simulink model "base_model_lqeH"  (R2020b)
settings: Solver=ode1  StartTime=0  StopTime=1150  FixedStep=0.1  RelTol=1e-3
libraries: simulink_extras x33
(part 2 of 3)

== matlab function base_model_lqeH/FormZ ==
  data: satInfo output size=[4,8]; satVisible input uint8 size=1; satCount input size=1; satCountPreset input; satVisibleFlag_GNSS input size=32; psdRange_sat input size=32; psdRange_INS input size=32; psdVel_INS input size=32; psdVel_sat input size=32; satNum output size=1; psdRange_INS_short output size=8; psdRange_GNSS_short output size=[8,1]; satVisibleFlag_INS input; satPosVel input; satPosVel_short output; dPsdRange input; sigmPsdRange output; satIDvis output uint8; satAzimutVis output; satEleavtionVis output; satAzimut input; satElevation input
function [satInfo, satNum, psdRange_INS_short, psdRange_GNSS_short, satPosVel_short, sigmPsdRange, satIDvis, satAzimutVis, satEleavtionVis] = ...
    getDGSK(satVisible, satCount, satCountPreset, satVisibleFlag_GNSS, psdRange_sat, ... 
    psdRange_INS,psdVel_INS, psdVel_sat, satVisibleFlag_INS, satPosVel, dPsdRange, satAzimut, satElevation)

    satCountPreset_fix = 20;
    
    satInfo             = zeros(4,8);
    psdRange_INS_short  = zeros(8,1);
    psdRange_GNSS_short = zeros(8,1);
    satPosVel_short     = zeros(6,8);
    sigmPsdRange        = zeros(8,1);
    
    satIDvis            = uint8(zeros(8,1));
    satAzimutVis        = zeros(8,1);
    satEleavtionVis     = zeros(8,1);
    
    satNum  = uint8(0);
    d_psdRange = 0;
    d_psdVel   = 0;
    for satID = 1:satCount
        
        if satVisibleFlag_GNSS(satID) == 1 && satVisibleFlag_INS(satID) == 1
            if satNum < satCountPreset
                satNum = satNum + 1;
            end
            d_psdRange = psdRange_INS(satID) - psdRange_sat(satID);
            d_psdVel   = psdVel_INS(satID)   - psdVel_sat(satID);
            
            satInfo(4,satNum) = psdRange_INS(satID);
            satIDvis(satNum)  = uint8(satID);
            
            
            satInfo(1,satNum) = satID;
            satInfo(2,satNum) = d_psdRange;
            satInfo(3,satNum) = d_psdVel;
            
            satAzimutVis(satNum)    = satAzimut(satID);
            satEleavtionVis(satNum) = satElevation(satID);
            
            satPosVel_short(:,satNum) = satPosVel(:,satID);
            
            sigmPsdRange(satNum) = dPsdRange(satID);
           
            
            psdRange_INS_short(satNum)  = psdRange_INS(satID);
            psdRange_GNSS_short(satNum) = psdRange_sat(satID);
        end      
    end
end

== matlab function base_model_lqeH/GNNS_freq_imitetor ==
  data: satNum_AV input size=1; satInfo output size=[4,8]; satInfo_AV input size=[4,8]; time_shift input size=1; satNum output uint8 size=1; timeDelay output size=1; frameAvalible_GNSS output uint8 size=1; satPosVel_AV input; satPosVel output; tStart input; tEnd input
function [satInfo, satNum, timeDelay, frameAvalible_GNSS,satPosVel]= getDGSK(satNum_AV, satInfo_AV, time_shift, satPosVel_AV, tStart, tEnd)

    satInfo   = zeros(4,8);
    satNum    = uint8(0);
    timeDelay = 0;
    satPosVel = zeros(6,8);

    GNSS_delay = 1;
    frameAvalible_GNSS = uint8(0);

    persistent time satInfo_mem satNum_mem satPosVel_mem timeInit

    if isempty(time)
        time = 0;
        timeInit = 0;
        
        satInfo_mem   = zeros(4,8);
        satNum_mem    = uint8(0);
        satPosVel_mem = zeros(6,8);
        
    end
    
    if timeInit > tStart
    
        if time > GNSS_delay
            satInfo_mem   = satInfo_AV  ; 
            satNum_mem    = satNum_AV   ;
            satPosVel_mem = satPosVel_AV;
            timeDelay     = time        ;
            time = 0;
            frameAvalible_GNSS = uint8(1);
        end

        timeDelay = GNSS_delay  ;
        satInfo   = satInfo_mem  ; 
        satNum    = satNum_mem   ;
        satPosVel = satPosVel_mem;

    %     satInfo(satErrNum) = satInfo(satErrNum) + psdErr;
    %     satInfo(1:3) = satInfo(1:3) + psdErr;

        time = time + time_shift;
    end
    timeInit = timeInit + time_shift;
end

== matlab function base_model_lqeH/GNSS_receiver_imitator6 ==
  data: alpha input; dyaw output; beta input; gamma input; heading input; pitch input; roll input; dpitch output; droll output; matr_CORR output
function [dyaw, dpitch,droll, matr_CORR] = GNSS_receiver_imitator (alpha, beta, gamma, heading, pitch, roll)

yaw = heading;
matr_CORR = zeros(3,3);
matrix = [sin(yaw)*tan(pitch), cos(yaw)*tan(pitch), -1;
          cos(yaw),           -sin(yaw),             0;
          sin(yaw)/cos(pitch), cos(yaw)/cos(pitch),  0];

dangles = [0;0;0];       

dangles = matrix*[alpha;beta;gamma];

dyaw   =  dangles(1);
dpitch =  dangles(2);
droll  =  dangles(3);
% 
% 
fix_heading = heading - dyaw;          
fix_pitch   = pitch   - dpitch;          
fix_roll    = roll    - droll;
% 
% matr_CORR = [ fix_heading,0,0;...
%              fix_pitch,0,0;...
%              fix_roll,0,0];
      
% matr_CORR =  [0 ,  gamma,-beta;...
%              -gamma, 0,  alpha;...
%               beta, -alpha, 0]; 

matr_CORR =  [ 0,       dyaw, -droll; ...
              -dyaw,    0,     dpitch;...
               droll, -dpitch, 0];

% matr_CORR =  [ dyaw, 0,      0; ...
%                0,    dpitch, 0;...
%                0,    0,      droll];







% if lqe_ctrl(1) == 1
%     mean_heading = circshift(mean_heading,-1);
%     mean_pitch   = circshift(mean_pitch,-1);
%     mean_roll    = circshift(mean_roll,-1);
% 
%     mean_heading(1) = dyaw;
%     mean_pitch(1)   = dpitch;
%     mean_roll(1)    = droll;
% 
% 
% end
% 
%     dyaw   = mean(mean_heading);
%     dpitch = mean(mean_pitch);
%     droll  = mean(mean_roll);


end

== matlab function base_model_lqeH/seter1 ==
  data: signal output size=1; time_shift input
function signal  = slowData(time_shift)
  
    persistent time_mem

    if isempty(time_mem)
        time_mem = 0;
    end
    
    signal = 0;
    time_mem = time_mem + time_shift;
    
    if time_mem >= 1
        signal = 1;
        time_mem = 0;
    end
    
end

== matlab function base_model_lqeH/DOPS ==
  data: PDOP output size=1; satPosVel input; HDOP output size=1; VDOP output size=1; TDOP output; satInfo input; psdRange_GNSS_short input size=[8,1]; satCountPreset input; posObj input; DOP output
function [PDOP, HDOP, VDOP,TDOP,DOP] = ...
    DOPS(satPosVel, satInfo, psdRange_GNSS_short, satCountPreset, posObj)

    PDOP = 0;
    HDOP = 0;
    VDOP = 0;
    TDOP = 0;
    DOP  = 0;
    matrixH = zeros(satCountPreset, 4);
    
%     satNum = 0;
    
    for ii = 1:satCountPreset
        if ii < length(satInfo(1,:))
            matrixH(ii, 1) = (satPosVel(1,ii) - posObj(1)) / psdRange_GNSS_short(ii);
            matrixH(ii, 2) = (satPosVel(2,ii) - posObj(2)) / psdRange_GNSS_short(ii);
            matrixH(ii, 3) = (satPosVel(3,ii) - posObj(3)) / psdRange_GNSS_short(ii);
            matrixH(ii, 4) = 1;
        end
    end
    
    Krt_2 = trace(inv(matrixH' * matrixH));
    
    
    Kr_2 = Krt_2 * 4/5;
    Kh_2 = Kr_2 * (1/((1/1.5 + 1)^2));
    
    DOP  = sqrt(Krt_2) ;
    PDOP = sqrt(Kr_2)  ; 
    TDOP = sqrt(Kr_2)/2;
    
    HDOP = sqrt(Kh_2)  ;
    VDOP = sqrt(Kh_2)*1.5;
    
    
    if  isnan(DOP)
        zz = 1;
    end
    
    
    
end

== matlab function base_model_lqeH/seter2 ==
  data: signal output size=1; time_shift input
function signal  = slowData(time_shift)
  
    persistent time_mem

    if isempty(time_mem)
        time_mem = 0;
    end
    
    signal = 0;
    time_mem = time_mem + time_shift;
    
    if time_mem >= 1
        signal = 1;
        time_mem = 0;
    end
    
end

== matlab function base_model_lqeH/Ve_err 1 ==
  data: data_out output size=1; data_in input; ctrl input
function data_out  = slowData(data_in, ctrl)
  
    persistent data_mem

    if isempty(data_mem)
        data_mem = data_in;
    end
    
    if ctrl == 1
        data_mem = data_in;
    end
    
    data_out = data_mem;
    
    
end

== matlab function base_model_lqeH/Fuck matlab5 ==
  data: satNum output; satVisible input; satIDs_fix output; psdRange_INSvis_fix output; psdRange_GNSSvis_fix output; satIDs input; baseSatID output; psdRange_INSvis input; psdRange_GNSSvis input; satCountPreset input
function [satNum, satIDs_fix,psdRange_INSvis_fix, psdRange_GNSSvis_fix, baseSatID]=  integrity_control(satVisible, satIDs, psdRange_INSvis, psdRange_GNSSvis, satCountPreset)
    
    %ограничивание числа спутников до satCountPreset = 8
    
    satIDs_fix           = zeros(8,1);
    psdRange_INSvis_fix  = zeros(8,1);
    psdRange_GNSSvis_fix = zeros(8,1);
    
    satNum = min([satVisible, satCountPreset]);
    
    for ii = 1:satVisible
        if ii <= satCountPreset
            satIDs_fix(ii) = satIDs(ii);
            psdRange_INSvis_fix (ii) = psdRange_INSvis(ii);
            psdRange_GNSSvis_fix(ii) = psdRange_GNSSvis(ii);
        end
    end

    baseSatID = satIDs(1);


end

== matlab function base_model_lqeH/Fuck matlab6 ==
  data: satAv output; satVisible input; satID_shrt input; satID_IC input
function satAv =  integrity_control(satVisible, satID_shrt, satID_IC)
    
    satAv = ones(8,1);
    persistent aa 
    if isempty(aa)
        aa = 0;
    end
        
    for ii = 1:8
        jj = find(satID_IC(ii) == satID_shrt);
        if ~isempty(jj)
            satAv(jj) = 0;
        end
    end


end

== matlab function base_model_lqeH/Fuck matlab7 ==
  data: psdRMiss output; size input
function psdRMiss =  integrity_control(size)
    
    psdRMiss = ones(8,1) .* size;

    
end

== matlab function base_model_lqeH/GNSS_integrity_control1 ==
  data: satNum input uint8 size=1; satID_in input; satAzimut_in input; satElevation_in input; psdRangeINS_in input; psdRangeGNSS_in input; baseSatID input uint8 size=1; satID_IC output uint8; intCtrl_status output uint8 size=1; lqe_F input; lqe_P input; lqe_L input; lqe_Q input; posObjINS input size=3; satPosVel input; lat input; lon input; alt input; disp_SatPos input; frameAvalible input; fastCritLevel output; fastLevel output; slowCritLevel output; satStartTime input; time_shift input; sensitivity input size=[4,1]; z_level output; z_crout output

function [satID_IC, intCtrl_status, fastCritLevel, fastLevel, slowCritLevel,...
          z_level, z_crout]=  integrity_control(satNum, satID_in, satAzimut_in, satElevation_in, ...
                                                         psdRangeINS_in, psdRangeGNSS_in, baseSatID,...                                                     
                                                         lqe_F, lqe_P, lqe_L, lqe_Q, posObjINS, satPosVel, lat, lon, alt, disp_SatPos, frameAvalible, satStartTime, time_shift, sensitivity)

    persistent intCtrl qq time
%--------------------------------------------------------------------------
%Константы
    disp_SatVel = 0.03;
    
    
    
    if isempty(intCtrl)
               
        qq = 0;
        time = 0;
        slowWindow = 600;% set max for code generation
        satLimit   = 8;
        
%         intCtrl.sensitivity = zeros(3,1);
        intCtrl.slowSensitivity = sensitivity(3);
        
        intCtrl.fastInit = uint8(0);
        intCtrl.psdRangeFast = zeros(satLimit,3);
        intCtrl.fastSatList = zeros(satLimit,1);
        
        
        intCtrl.slowInit = uint8(0);
        intCtrl.psdRangeSlow = ones(slowWindow,satLimit);
        intCtrl.slowSatList  = zeros(satLimit,1);
        
        intCtrl.probSatID = uint8(zeros(satLimit,1));
        intCtrl.moniSatID = uint8(zeros(satLimit,1));
        
        intCtrl.probSatNum = uint8(0);
        intCtrl.moniSatNum = uint8(0);
        
        intCtrl.baseSatID = uint8(0);
        
        intCtrl.satLossFrame     = zeros(satLimit,2); %Строка 1 не задейстоввана?
        intCtrl.satLossFrameAlow = uint8(10);
        
        intCtrl.slowMean = zeros(satLimit,2);
        intCtrl.slowDisp = zeros(satLimit,1);
        
        intCtrl.fastExpt = zeros(satLimit,1);%Не задействовано
        
        intCtrl.fastExptCriteria = zeros(satLimit,2);
        
        intCtrl.criteriaScale = ones(2,1) .* [sensitivity(1); sensitivity(2)]; 
        
        intCtrl.slowWindow      = slowWindow;
        intCtrl.slowWindow_size = sensitivity(4);
        intCtrl.satLimit        = satLimit;
    end
%--------------------------------------------------------------------------
%Объявление выходых параметров 
    satID_IC       = uint8(zeros(8 ,1));%uint8(zeros(intCtrl.satLimit ,1));
    fastCritLevel  =       zeros(8,1);%zeros(intCtrl.satLimit ,1);
    fastLevel      =       zeros(8,1);%zeros(intCtrl.satLimit ,1);
    slowCritLevel  =       zeros(8,1);%zeros(intCtrl.satLimit ,1);
    intCtrl_status =       uint8(1); %%uint8(1); %
    z_crout        =       zeros(1,1);%zeros(1,1);
    z_level        =       zeros(8,1);%zeros(intCtrl.satLimit ,1);
    
%--------------------------------------------------------------------------
%Костыль для подержания много спутников (Если всегда +- 8 но подскакивает до 12)

    satID        = uint8(zeros(intCtrl.satLimit,1));
    satAzimut    =       zeros(intCtrl.satLimit,1);
    satElevation =       zeros(intCtrl.satLimit,1);
    psdRangeINS  =       zeros(intCtrl.satLimit,1);
    psdRangeGNSS =       zeros(intCtrl.satLimit,1);
    
    for ii = 1:satNum
        satID(ii)        = satID_in(ii);
        satAzimut(ii)    = satAzimut_in(ii);
        satElevation(ii) = satElevation_in(ii);
        psdRangeINS(ii)  = psdRangeINS_in(ii);
        psdRangeGNSS(ii) = psdRangeGNSS_in(ii);
    end

%--------------------------------------------------------------------------  
%Обновление ID базового спутника
    intCtrl.baseSatID = baseSatID;
%--------------------------------------------------------------------------
%Счетчик пропущенных измерений НКА. Для "рабочих" НКА, счетчик обнуляется 
    intCtrl.satLossFrame(:,2) = intCtrl.satLossFrame(:,2) + 1;
    for ii = 1:satNum
        if find(satID(ii) == intCtrl.satLossFrame(:,1))
            intCtrl.satLossFrame(ii,2) = 0;
        end
    end
%--------------------------------------------------------------------------
    if frameAvalible == 1                                                  %Ждать поступления измерения псевдодальности
                                                                           %Быстрый цикл  
%                                                                          Набор информации (первых и вторых разностей)
        intCtrl = fastCircle (intCtrl, satNum, satID, psdRangeGNSS, psdRangeINS, disp_SatPos,...
                              lqe_F, lqe_P, lqe_L, lqe_Q, lat, lon, alt, posObjINS, satPosVel, disp_SatVel);
                                                                            %Набор информации (первых разностей)
                                                                           %Проверка по критерию
        probSatCount = 0;
        %intCtrl.probSatID = uint8(zeros(intCtrl.satLimit,1));%
        intCtrl.probSatID = uint8(zeros(8,1));
        for ii = 1:satNum
            if abs(intCtrl.psdRangeFast(ii,3)) >= (intCtrl.fastExptCriteria(ii))
                probSatCount = probSatCount + 1;
                intCtrl.probSatID(probSatCount) = satID(ii);
            end
        end
                                                                            %Медленный цикл  
                                                                            %Набор информации (вторых разностей и среднего)
    intCtrl = slowCircleLogic(intCtrl, satNum, satID, psdRangeGNSS, psdRangeINS);
%     
    
    for ii = 1:satNum
        baseMean = 0;
        baseDisp = intCtrl.slowDisp(ii);
%         alpha = intCtrl.slowSensitivity;
%         Z = (intCtrl.slowMean(ii) -  baseMean) ./ sqrt(intCtrl.slowDisp(ii) * 2/intCtrl.slowWindow(1:intCtrl.slowWindow_size));
%may be ERROR        
        Z = (intCtrl.slowMean(ii) -  baseMean) ./ sqrt(intCtrl.slowDisp(ii) * 2/intCtrl.slowWindow_size);
%         Z_criteria = tinv(1 - intCtrl.slowSensitivity, intCtrl.slowWindow(1:intCtrl.slowWindow_size) - 2 - 1);
        Z_criteria = tinv(intCtrl.slowSensitivity, intCtrl.slowWindow_size - 2 - 1);%(1:intCtrl.slowWindow_size)
        z_level(ii) = abs(Z);
        z_crout = Z_criteria;
   %Slow circle decision-making segment
        if abs(Z) >= Z_criteria
            jj = find(satID(ii) == intCtrl.probSatID);
            if length(jj) == 0
                probSatCount = probSatCount + 1;        
                intCtrl.probSatID(probSatCount) = satID(ii);  
                qq = qq + 1;
                if qq == 900
                    tt = 1;
                end
            end
        end
    end
    
    end
    
fastLevel     = abs(intCtrl.psdRangeFast(:,3));    
fastCritLevel = intCtrl.fastExptCriteria(:,1);
slowCritLevel = abs(intCtrl.slowMean(:,1));
% z_level = abs(Z);
% z_crout = Z_criteria;

%--------------------------------------------------------------------------
    
%--------------------------------------------------------------------------
                                                                            %Отбор спутников и формирование выходной информации
                                                                     
    id = 0;
    intCtrl_status = uint8(1);% 1 - IC pass; 0 - IC fault
    time = time + time_shift;
%     if time > (satStartTime + intCtrl.slowWindow(1:intCtrl.slowWindow_size) * 4) 
    if time > (satStartTime + intCtrl.slowWindow_size * 4)%(1:intCtrl.slowWindow_size)
        for ii = 1:satNum
            if find(satID(ii) == intCtrl.probSatID)
                id = id + 1;
                satID_IC(id) = satID(ii);
            end
        end
        if satNum - id <= 4  
            intCtrl_status = uint8(0);
        end
    end
    
end


%==========================================================================
function [D_rho, D_rho_dot] = fastCriteriaMath( a,e2,C,Ro_mark,R_tp,disp_SatPos_mem, ...
                                    ii,lat,lon,alt, psdRange,posObj, satPosVel,...
                                    disp_SatPos, disp_SatVel)
        
        
        dPsdRange_dLambda =  (1/psdRange(ii)) * (Ro_mark + alt)*cos(lat)*...
                                                (sin(lon)*(satPosVel(1,ii) - posObj(1)) - ...
                                                 cos(lon)*(satPosVel(2,ii) - posObj(2)));

        dPsdRange_dphi    =  (1/psdRange(ii))   * ...
                              ((satPosVel(1,ii) - posObj(1)) * (- cos(lon) * cos(lat) * R_tp + (Ro_mark + alt) * cos(lon) * sin(lat)) + ...%dRz_dLat
                               (satPosVel(2,ii) - posObj(2)) * (- sin(lon) * cos(lat) * R_tp + (Ro_mark + alt) * sin(lon) * sin(lat)) + ...%dRz_dLat
                               (satPosVel(3,ii) - posObj(3)) * (- (1 - e2) * sin(lat) * R_tp - ((1 - e2) * Ro_mark + alt) * cos(lat)));    %dRz_dLat

        dPsdVel_dot_dVe   =  (1/psdRange(ii)) * (...
                                sin(lon) * (satPosVel(1,ii) - posObj(1)) - ...
                                cos(lon) * (satPosVel(2,ii) - posObj(2)));

        dPsdVel_dot_dVn   =  (1/psdRange(ii)) * (...
                                cos(lon)*sin(lat)*(satPosVel(1,ii) - posObj(1)) + ...
                                sin(lon)*sin(lat)*(satPosVel(2,ii) - posObj(2)) - ...
                                cos(lat)*         (satPosVel(3,ii) - posObj(3)));

        dPsdRange_dAlt    = (-1/psdRange(ii))* (...
                                cos(lat)*cos(lon)*(satPosVel(1,ii) - posObj(1)) + ...
                                cos(lat)*sin(lon)*(satPosVel(2,ii) - posObj(2)) + ...
                                sin(lat)*         (satPosVel(3,ii) - posObj(3)));
%--------------------------------------------------------------------------
%Формирование дисперсий
        dPsdVel_dot_dVh   = (-1/psdRange(ii))* (...
                                cos(lon)*cos(lat)*(satPosVel(1,ii) - posObj(1)) + ...
                                sin(lon)*cos(lat)*(satPosVel(2,ii) - posObj(2)) + ...
                                sin(lat)*         (satPosVel(3,ii) - posObj(3)));
%--------------------------------------------------------------------------
%Пересчет из радиан в метры
                            
        ro_1 = a*(1-e2)/(1-e2*sin(lat)^2)^(3/2) + alt;
        ro_2 = a*(1-e2*sin(lat)^2)^(-1/2) + alt;                      
        dPsdRange_dLambda =  (1/(ro_2 * cos(lat))) * dPsdRange_dLambda;
        dPsdRange_dphi    =  (1/ro_1) * dPsdRange_dphi;                 
%--------------------------------------------------------------------------
        D_hor = sum(abs([dPsdRange_dLambda, dPsdRange_dphi ]) * [C(1,1), C(1,2) ;...
                                                            C(2,1), C(2,2)]);
        D_vel = sum(abs([dPsdVel_dot_dVe,   dPsdVel_dot_dVn]) * [C(3,3), C(3,4) ;...
                                                            C(4,3), C(4,4)]);    
                                                        
        D_alt  = abs(dPsdRange_dAlt)  * C(20,20);
        D_vAlt = abs(dPsdVel_dot_dVh) * C(21,21);


        D_rho     = D_hor + D_alt  + disp_SatPos + disp_SatPos_mem;
        D_rho_dot = D_vel + D_vAlt + 2*disp_SatVel;

end



function intCtrl = fastCircle(intCtrl, satNum, satID, psdRangeGNSS, psdRangeINS, disp_SatPos,...
                              lqe_F, lqe_P, lqe_L, lqe_Q, lat, lon, alt, posObjINS, satPosVel, disp_SatVel)
    
    persistent disp_SatPos_mem

    if isempty(disp_SatPos_mem)
        disp_SatPos_mem = zeros(size(disp_SatPos));
        disp_SatPos_mem = disp_SatPos;
    end

%--------------------------------------------------------------------------
%Константы    
    a = 6378136;
    e2 = 0.0066943662;
%--------------------------------------------------------------------------
%Матрица связи С (?)        
    C = lqe_F*lqe_P*lqe_F' + lqe_L*lqe_Q*lqe_L' + lqe_P + 2*lqe_F*lqe_P;
    Ro_mark = a / sqrt(1 - e2*(sin(lat))^2);
%--------------------------------------------------------------------------
%Коэффициенты (направляющие косинусы). Аналагично матрице связи Н (ЖСК)        
    
    dRz_dLat = a*e2*cos(lat)*sin(lat) / ((1 - e2*sin(lat)^2)^(3/2));
    R_tp     = sin(lat)*(a + alt) - cos(lat)*dRz_dLat;  

    if intCtrl.fastInit == 0
        for ii = 1:satNum
            intCtrl.psdRangeFast(ii, 1) = 1;%(psdRangeGNSS(ii) - psdRangeGNSS(intCtrl.baseSatID));
            intCtrl.psdRangeFast(ii, 2) = intCtrl.psdRangeFast(ii, 1);
            intCtrl.fastSatList(ii)     = satID(ii);
            intCtrl.fastInit            = uint8(1); 
        end
    end


    for ii = 1:satNum
        sID = find(satID(ii) == intCtrl.fastSatList);%Был ли этот спутник раньше
        if ~isempty(sID) %Если этот спутник уже есть и обрабатывается 
            
            thirdDifference_previous = intCtrl.psdRangeFast(sID, 1);
            intCtrl.psdRangeFast(sID, 1) = psdRangeGNSS(sID) - psdRangeINS(sID);
            intCtrl.psdRangeFast(sID, 3) = intCtrl.psdRangeFast(sID, 1) - thirdDifference_previous;                                               
%             
            [D_rho, D_rho_dot] = fastCriteriaMath( a,          e2,        C,  Ro_mark,      R_tp, disp_SatPos_mem(ii), ...
                                                  ii,      lat,      lon,       alt, psdRangeINS,   posObjINS, satPosVel, disp_SatPos(ii), disp_SatVel);
                                                  
            intCtrl.fastExptCriteria(sID,1) = intCtrl.criteriaScale(1) * sqrt(abs(D_rho)    );
            intCtrl.fastExptCriteria(sID,2) = intCtrl.criteriaScale(2) * sqrt(abs(D_rho_dot));
        
        else % Если появился спутник
            if ii <= intCtrl.satLimit % Если не превышен лимит н спутники
                if length(find(intCtrl.fastSatList == 0)) ~= 0% Если есть слоты для спутников
                    %------Инициализация
                    sID = find(intCtrl.fastSatList == 0, 1,'first');% Вязть первый пустой слот
                    intCtrl.fastSatList (sID)    = satID(ii);% Записать ID нового спутника
                    
                    %--------------------------------------
                    %Замена на 3 разности
                            thirdDifference_previous = intCtrl.psdRangeFast(sID, 1);
                            intCtrl.psdRangeFast(sID, 1) = psdRangeGNSS(sID) - psdRangeINS(sID);
                            intCtrl.psdRangeFast(sID, 3) = intCtrl.psdRangeFast(sID, 1) - thirdDifference_previous;  
                    
                  
                    [D_rho, D_rho_dot] = fastCriteriaMath(   a,          e2,        C, dRz_dLat,      R_tp, disp_SatPos_mem(ii), ...
                                                            ii,      lat,      lon,       alt, psdRangeINS,   posObjINS, satPosVel, disp_SatPos(ii), disp_SatVel);                           
                    intCtrl.fastExptCriteria(sID,1) = intCtrl.criteriaScale(1) * sqrt(abs(D_rho)    );
                    intCtrl.fastExptCriteria(sID,2) = intCtrl.criteriaScale(2) * sqrt(abs(D_rho_dot));
                    
                else % Если нет слотов
                    jj = find(intCtrl.satLossFrame(:,2) >= intCtrl.satLossFrameAlow, 1, 'first');%Найти просрочку
                    if ~isempty(jj)% Если есть просроченые спутники
                    %------Инициализация
                        intCtrl.fastSatList(jj)     = satID(ii);
                    %--------------------------------------
                    %Замена на 3 разности
                            thirdDifference_previous = intCtrl.psdRangeFast(sID, 1);
                            intCtrl.psdRangeFast(sID, 1) = psdRangeGNSS(sID) - psdRangeINS(sID);
                            intCtrl.psdRangeFast(sID, 3) = intCtrl.psdRangeFast(sID, 1) - thirdDifference_previous; 
                        
                                   
                        [D_rho, D_rho_dot] = fastCriteriaMath(	 a,          e2,        C, dRz_dLat,       R_tp, disp_SatPos_mem(ii), ...
                                                                ii,      lat,      lon,       alt, psdRangeINS,   posObjINS, satPosVel, disp_SatPos(ii), disp_SatVel);
                                                  
                        intCtrl.fastExptCriteria(sID,1) = intCtrl.criteriaScale(1) * sqrt(abs(D_rho)    );
                        intCtrl.fastExptCriteria(sID,2) = intCtrl.criteriaScale(2) * sqrt(abs(D_rho_dot));
                    end
                end
            end
        end
        
        
    end
    
end








function intCtrl = slowCircleLogic(intCtrl, satNum, satID, psdRangeGNSS, psdRangeINS)

%--------------------------------------------------------------------------
%Инициализация
    if intCtrl.slowInit == 0
        for ii = 1:satNum
            intCtrl.slowSatList(ii)    = satID(ii);
%             intCtrl.psdRangeSlow(:,ii) = intCtrl.psdRangeSlow(:,ii) .*...
%                 ((psdRangeGNSS(ii)                   - psdRangeINS(ii))     ...
%                - (psdRangeGNSS(intCtrl.baseSatID) - psdRangeINS(intCtrl.baseSatID)));
        end
        intCtrl.slowInit = uint8(1);
    end
%--------------------------------------------------------------------------
%Медленный цикл
    for ii = 1:satNum
%         if find(satID(ii) ~= intCtrl.probSatID)
        if find(satID(ii) == intCtrl.slowSatList) %Если спутник уже был
            intCtrl = slowCircleAction(intCtrl, ii, psdRangeGNSS(ii), psdRangeINS(ii)); %обработка
        else 
            if length(find(intCtrl.slowSatList == 0)) ~= 0% Если есть слоты для спутников
                %------Инициализация
                sID = find(intCtrl.slowSatList == 0, 1,'first');% Взять первый пустой слот
                intCtrl.slowSatList(sID) = satID(ii);
                %max set only here
                intCtrl.psdRangeSlow((1:intCtrl.slowWindow_size),sID) = ones(uint16(intCtrl.slowWindow_size),1).*...
                                                 (psdRangeGNSS(ii)                - psdRangeINS(ii));% - ...
                                                  %(psdRangeGNSS(intCtrl.baseSatID) - psdRangeINS(intCtrl.baseSatID)));
                intCtrl = slowCircleAction(intCtrl, sID, psdRangeGNSS(ii), psdRangeINS(ii));
                fkngtest = 1;
            else % Если нет слотов
                jj = find(intCtrl.satLossFrame(:,2) >= intCtrl.satLossFrameAlow, 1, 'first');%Найти просрочку
                if ~isempty(jj)% Если есть просроченые спутники
                %------Инициализация
                    intCtrl.slowSatList(jj) = satID(ii);
                    intCtrl.psdRangeSlow((1:intCtrl.slowWindow_size),jj) = ones(uint16(intCtrl.slowWindow_size),1).*...
                                                    (psdRangeGNSS(ii)                - psdRangeINS(ii));
                    intCtrl = slowCircleAction(intCtrl, jj, psdRangeGNSS(ii), psdRangeINS(ii));
                end
            end
        end
            
            
            
            
            
%             if ii <= intCtrl.satLimit %Если не превышено количество спутников
%                 jj = find(intCtrl.satLossFrame(:,2) >= intCtrl.satLossFrameAlow, 1, 'first');% 
%                 intCtrl.slowSatList(jj) = satID(ii);
% 
%                 intCtrl.psdRangeSlow(:,jj) = ones(intCtrl.slowWindow(1:slowWindow_size),1).*...
%                                                 ((psdRangeGNSS(ii)                - psdRangeINS(ii))...
%                                                - (psdRangeGNSS(intCtrl.baseSatID) - psdRangeINS(intCtrl.baseSatID)));
% 
%                 intCtrl = slowCircleAction(intCtrl, jj, psdRangeGNSS, psdRangeINS);
%             end
%         end
%         end
    end
end

function intCtrl = slowCircleAction(intCtrl, id, psdRangeGNSS, psdRangeINS)

    intCtrl.psdRangeSlow(1:intCtrl.slowWindow_size,id) = circshift(intCtrl.psdRangeSlow(1:intCtrl.slowWindow_size,id),1);
    intCtrl.psdRangeSlow(1,id) = (psdRangeGNSS - psdRangeINS);
   %intCtrl.psdRangeSlow(1,id) = (psdRangeGNSS(id) - psdRangeINS(id)) - (psdRangeGNSS(intCtrl.baseSatID) - psdRangeINS(intCtrl.baseSatID));  
    intCtrl.psdRangeSlow(1,id) = intCtrl.psdRangeSlow(1,id) - intCtrl.slowMean(id,2);
    intCtrl.slowMean(id,2)     = (psdRangeGNSS - psdRangeINS);
    
    
    intCtrl.slowMean(id,1)= mean(intCtrl.psdRangeSlow(1:intCtrl.slowWindow_size,id));
    intCtrl.slowDisp(id)  =  std(intCtrl.psdRangeSlow(1:intCtrl.slowWindow_size,id));
end

== matlab function base_model_lqeH/Fuck matlab8 ==
  data: corruptValue output; tStart input; tp input; tEnd input; errSize input; corruptTimeStart input; corruptPSDError input; corruptErrorType input; dt input
function corruptValue = integrity_control(tStart, tp, tEnd, errSize,...
                    corruptTimeStart, corruptPSDError, corruptErrorType, dt)
%chouse psd error type
    persistent time
    if isempty(time)  
        time = 0;
    end
    corruptValue = 0;
    if time >= corruptTimeStart
        
        if corruptErrorType == 1
            corruptValue = corruptPSDError;
        elseif corruptErrorType == 2
            corruptValue = corruptPSDError * (time - corruptTimeStart);
        else
            corruptValue = 0;
        end
    end

    time = time + dt;


    % %--------------------------------------------------------------------------
    % if time > tStart && time < tp 
    %      time_out = errSize;%*(time-tStart);%time - tStart;
    % end
    % 
    % 
    % if time > tp && time < tEnd
    %     time_out = 0;%*(time-tStart);%time - tStart;
    % end
    % 
    % if time > tEnd
    %     time_out = -errSize;%*(time-tStart);%time - tStart;
    % end
    % 
    % if tStart < time && tp > time
    %      time_out = errSize;%*(time-tStart);%time - tStart;
    % end
    % 




    % % --------------------------------------------------------------------------
%     if tStart < time
%         time_out = errSize*(time-tStart);%time - tStart;
%     end
    % % 




end

== matlab function base_model_lqeH/Fuck matlab9 ==
  data: satID_forCtrl output; satID_IC input
function satID_forCtrl =  forCtrl(satID_IC)
    

    satID_forCtrl = satID_IC(1:3);
    
    
end

== matlab function base_model_lqeH/Fuck matlab10 ==
  data: psdRange_fix output; satID input; psdRangeSat input; satCoefs input; satInctrl input
function psdRange_fix =  integrity_control(satID, psdRangeSat, satCoefs, satInctrl)
    


    psdRange_fix = psdRangeSat;

    for ii = 1:3
        jj = find(satInctrl(ii) == satID);
        psdRange_fix(jj) = psdRangeSat(jj) - satCoefs(1,ii) - satCoefs(2,ii) * satCoefs(4,ii) - satCoefs(3,ii) * satCoefs(4,ii).^2;
    end
    

end

== matlab function base_model_lqeH/altimetrImitator ==
  data: alt_ideal input; Vh input; Alt output; RMS output; isAltAvalible output; timeStep output; time_shift input
function [Alt, RMS, isAltAvalible, timeStep] = altimetrImitator(alt_ideal, Vh, time_shift)
        
Alt = 0;
RMS = 1000;
isAltAvalible = 0;
timeStep = 0;


%     persistent timer altMem rH
%     if isempty(timer)
%         altMem = alt_ideal;
%         timer        = 0;
%         rng(0,'twister');
%         rH = 100;
%     end     
%     
%     timeStep_fix = 0.7;%установка частоты выдачи данных
%     deltaH = 0.02;
%     rH0 = 1;
%     Alt = 0;
%     RMS = 100;
%     isAltAvalible = 0;
%     timeStep = 0.7;
%     
%     if timer > timeStep_fix
%         if alt_ideal < 5000
%             H_dot = alt_ideal - altMem;
%             altMem = alt_ideal;
%             rH = deltaH*H_dot.^2 + rH0;
%             Alt = alt_ideal + rH*randn()/5;
%             isAltAvalible = 1;
%             timeStep = timer;
%         end
%         timer = 0;
%     else
%         timer = timer + time_shift;    
%     end
%     
%     RMS = rH;

end

== matlab function base_model_lqeH/GNSS_receiver_imitator7 ==
  data: satCoefs input; sat1_id output; sat1_a output; sat1_b output; sat1_c output; sat1_t output; satInctrl input
function [sat1_id, sat1_a,sat1_b, sat1_c, sat1_t] = GNSS_receiver_imitator (satCoefs,satInctrl)

sat1_id  = satInctrl(1);
sat1_a   = satCoefs(1,1);
sat1_b   = satCoefs(2,1);
sat1_c   = satCoefs(3,1);
sat1_t   = satCoefs(4,1);

end

== matlab function base_model_lqeH/GNSS_receiver_imitator8 ==
  data: satCoefs input; sat1_id output; sat1_cfs output; satInctrl input
function [sat1_id, sat1_cfs] = GNSS_receiver_imitator (satCoefs,satInctrl)

sat1_id       = satInctrl(1);
sat1_cfs      = zeros(4,1);
sat1_cfs(1,1) = satCoefs(1,1);
sat1_cfs(2,1) = satCoefs(2,1);
sat1_cfs(3,1) = satCoefs(3,1);
sat1_cfs(4,1) = satCoefs(4,1);

end

== matlab function base_model_lqeH/GNSS_receiver_imitator9 ==
  data: satCoefs input; sat1_id output; sat1_cfs output; satInctrl input
function [sat1_id, sat1_cfs] = GNSS_receiver_imitator (satCoefs,satInctrl)

sat1_id       = satInctrl(2);
sat1_cfs      = zeros(4,1);
sat1_cfs(1,1) = satCoefs(1,2);
sat1_cfs(2,1) = satCoefs(2,2);
sat1_cfs(3,1) = satCoefs(3,2);
sat1_cfs(4,1) = satCoefs(4,2);

end

== matlab function base_model_lqeH/GNSS_receiver_imitator10 ==
  data: satCoefs input; sat1_id output; sat1_cfs output; satInctrl input
function [sat1_id, sat1_cfs] = GNSS_receiver_imitator (satCoefs,satInctrl)

sat1_id       = satInctrl(2);
sat1_cfs      = zeros(4,1);
sat1_cfs(1,1) = satCoefs(1,3);
sat1_cfs(2,1) = satCoefs(2,3);
sat1_cfs(3,1) = satCoefs(3,3);
sat1_cfs(4,1) = satCoefs(4,3);

end

== matlab function base_model_lqeH/Vh_err 1 ==
  data: data_out output size=1; data_in input; ctrl input
function data_out  = slowData(data_in, ctrl)
  
    persistent data_mem

    if isempty(data_mem)
        data_mem = data_in;
    end
    
    if ctrl == 1
        data_mem = data_in;
    end
    
    data_out = data_mem;
    
    
end

== matlab function base_model_lqeH/Vn_err 1 ==
  data: data_out output size=1; data_in input; ctrl input
function data_out  = slowData(data_in, ctrl)
  
    persistent data_mem

    if isempty(data_mem)
        data_mem = data_in;
    end
    
    if ctrl == 1
        data_mem = data_in;
    end
    
    data_out = data_mem;
    
    
end

== matlab function base_model_lqeH/alt_err 1 ==
  data: data_out output size=1; data_in input; ctrl input
function data_out  = slowData(data_in, ctrl)
  
    persistent data_mem

    if isempty(data_mem)
        data_mem = data_in;
    end
    
    if ctrl == 1
        data_mem = data_in;
    end
    
    data_out = data_mem;
    
    
end

== matlab function base_model_lqeH/bigHeadingFix2 ==
  data: headingError input; fix_headingError output
function fix_headingError  = fix2PIerr (headingError)

    fix_headingError = headingError;
    if headingError > 0.95*(3.1415)
        fix_headingError = -2*3.1415 + headingError;
    end
% 
% 
%     persistent headingError_mem
%     if isempty(headingError_mem)
%         headingError_mem = headingError;
%     end
%     fix_headingError = headingError;
%     if abs(fix_headingError) > 0.95*(2*3.1415)
%         fix_headingError = headingError_mem;
%     else
%         headingError_mem = headingError;    
%     end
end

== matlab function base_model_lqeH/coord_err7 ==
  data: dlat input; x output; dlon input; lat input; y output; alt input
function [x, y]= GNSS_receiver_imitator (dlat, dlon, lat, alt)
    
    height = 0;
    
    beta  = 0.0053171;
    beta1 = 71*10^-7;
    q  = 0.00346775;
    ge = 9.78049;
    a = 6378136;                                                           %PZ-90
    e2 = 0.0066943662; 


    ro_1 = a*(1-e2)/(1-(e2)*(sin(lat)^2))^(3/2) + alt;
    ro_2 = a/((1-(e2)*(sin(lat)^2))^(1/2)) + alt;

%EARTH_A = 6378147;
     x  = dlat*(ro_1);                            %d_longitude
     y  = dlon*(ro_2*cos(lat));    
end

== matlab function base_model_lqeH/coord_err8 ==
  data: dlat input; x output; dlon input; lat input; y output; alt input
function [x, y]= GNSS_receiver_imitator (dlat, dlon, lat, alt)
    persistent X_mem Y_mem
    if isempty(X_mem)
        Y_mem = dlat;
        X_mem = dlon;
    end
%     height = 0;
    
    beta  = 0.0053171;
    beta1 = 71*10^-7;
    q  = 0.00346775;
    ge = 9.78049;
    a = 6378136;                                                           %PZ-90
    e2 = 0.0066943662; 


    ro_1 = a*(1-e2)/(1-(e2)*(sin(lat)^2))^(3/2) + alt;
    ro_2 = a/((1-(e2)*(sin(lat)^2))^(1/2)) + alt;

%EARTH_A = 6378147;
     x  = (dlat - Y_mem)*(ro_1);                            %d_longitude
     y  = (dlon - X_mem)*(ro_2*cos(lat));    
end

== matlab function base_model_lqeH/altimetrImitator1 ==
  data: psdRangeNoise input; PDOP input; HDOP input; VDOP input; sigmPsdRange output; TDOP input; sigmPsdVel output; timeStep input
function [sigmPsdRange, sigmPsdVel] = altimetrImitator(psdRangeNoise, PDOP, HDOP, VDOP, TDOP,timeStep)

%     persistent time_mem
%     if isempty(time_mem)
%         time_mem = 0;
%     end

    sigmCrd = 6;
    sigmVel = 0.2;
%     time_mem = time_mem + timeStep;
%     if time_mem  < 150 
% %         sigmCrd = sigmCrd*3;
%         sigmVel = sigmVel*3;
%     end

%     sigmPsdRange = ones(8,1).*sigmCrd./PDOP;
    sigmPsdVel   = ones(8,1).*sigmVel./VDOP;

    sigmPsdRange = ones(8,1) * mean(psdRangeNoise);

end

== matlab function base_model_lqeH/heading_INS  1 ==
  data: headingError input; fix_headingError output
function fix_headingError  = fix2PIerr (headingError)

    persistent headingError_mem
    if isempty(headingError_mem)
        headingError_mem = headingError;
    end
    fix_headingError = headingError;
    if abs(fix_headingError) > 0.95*(360)
        fix_headingError = headingError_mem;
    else
        headingError_mem = headingError;    
    end
end

== matlab function base_model_lqeH/heading_INS  2 ==
  data: headingError input; fix_headingError output
function fix_headingError  = fix2PIerr (headingError)

    persistent headingError_mem
    if isempty(headingError_mem)
        headingError_mem = headingError;
    end
    fix_headingError = headingError;
    if abs(fix_headingError) > 0.95*(360)
        fix_headingError = headingError_mem;
    else
        headingError_mem = headingError;    
    end
end

== matlab function base_model_lqeH/heading_err      ==
  data: data_out output size=1; data_in input; ctrl input
function data_out  = slowData(data_in, ctrl)
  
    persistent data_mem

    if isempty(data_mem)
        data_mem = data_in;
    end
    
    if ctrl == 1
        data_mem = data_in;
    end
    
    data_out = data_mem;
    
    
end

== matlab function base_model_lqeH/heading_err     1 ==
  data: data_out output size=1; data_in input; ctrl input
function data_out  = slowData(data_in, ctrl)
  
    persistent data_mem

    if isempty(data_mem)
        data_mem = data_in;
    end
    
    if ctrl == 1
        data_mem = data_in;
    end
    
    data_out = data_mem;
    
    
end

== matlab function base_model_lqeH/heading_err     2 ==
  data: data_out output size=1; data_in input; ctrl input
function data_out  = slowData(data_in, ctrl)
  
    persistent data_mem

    if isempty(data_mem)
        data_mem = data_in;
    end
    
    if ctrl == 1
        data_mem = data_in;
    end
    
    data_out = data_mem;
    
    
end

== matlab function base_model_lqeH/heading_err     3 ==
  data: data_out output size=1; data_in input; ctrl input
function data_out  = slowData(data_in, ctrl)
  
    persistent data_mem

    if isempty(data_mem)
        data_mem = data_in;
    end
    
    if ctrl == 1
        data_mem = data_in;
    end
    
    data_out = data_mem;
    
    
end

== matlab function base_model_lqeH/heading_err     4 ==
  data: data_out output size=1; data_in input; ctrl input
function data_out  = slowData(data_in, ctrl)
  
    persistent data_mem

    if isempty(data_mem)
        data_mem = data_in;
    end
    
    if ctrl == 1
        data_mem = data_in;
    end
    
    data_out = data_mem;
    
    
end

== matlab function base_model_lqeH/heading_err  1 ==
  data: headingError input; fix_headingError output
function fix_headingError  = fix2PIerr (headingError)

    persistent headingError_mem
    if isempty(headingError_mem)
        headingError_mem = headingError;
    end
    fix_headingError = headingError;
    if abs(fix_headingError) > 0.99*(360)
        fix_headingError = headingError_mem;
    else
        headingError_mem = headingError;    
    end
end

== matlab function base_model_lqeH/heading_err_FBon 2 ==
  data: headingError input; fix_headingError output
function fix_headingError  = fix2PIerr (headingError)

    persistent headingError_mem
    if isempty(headingError_mem)
        headingError_mem = headingError;
    end
    fix_headingError = headingError;
    if abs(fix_headingError) > 0.95*(2*3.1415)
        fix_headingError = headingError_mem;
    else
        headingError_mem = headingError;    
    end
end

== matlab function base_model_lqeH/lat_err 1 ==
  data: data_out output size=1; data_in input; ctrl input
function data_out  = slowData(data_in, ctrl)
  
    persistent data_mem

    if isempty(data_mem)
        data_mem = data_in;
    end
    
    if ctrl == 1
        data_mem = data_in;
    end
    
    data_out = data_mem;
    
    
end

== matlab function base_model_lqeH/lon_err 1 ==
  data: data_out output size=1; data_in input; ctrl input
function data_out  = slowData(data_in, ctrl)
  
    persistent data_mem

    if isempty(data_mem)
        data_mem = data_in;
    end
    
    if ctrl == 1
        data_mem = data_in;
    end
    
    data_out = data_mem;
    
    
end

== matlab function base_model_lqeH/pitch_err     ==
  data: data_out output size=1; data_in input; ctrl input
function data_out  = slowData(data_in, ctrl)
  
    persistent data_mem

    if isempty(data_mem)
        data_mem = data_in;
    end
    
    if ctrl == 1
        data_mem = data_in;
    end
    
    data_out = data_mem;
    
    
end

== matlab function base_model_lqeH/roll_err      ==
  data: data_out output size=1; data_in input; ctrl input
function data_out  = slowData(data_in, ctrl)
  
    persistent data_mem

    if isempty(data_mem)
        data_mem = data_in;
    end
    
    if ctrl == 1
        data_mem = data_in;
    end
    
    data_out = data_mem;
    
    
end

== matlab function base_model_lqeH/ADD error SAT ==
  data: satInfo input; psdRange_spuff output; LQE_Z_spuff output; corruptSatCount input; psdRange_SATvis input; errVal input; satID input; satCoefs input; satInctrl input; ctrlSatCoefs input
function [psdRange_spuff, LQE_Z_spuff] =  AddingDivertingHindrance(satInfo, corruptSatCount, psdRange_SATvis, errVal,...
                                                                   satID, satCoefs, satInctrl, ctrlSatCoefs)
   %add psd error here
   
    psdRange_spuff = zeros(8,1);
    psdRange_spuff = psdRange_SATvis;
    
    LQE_Z_spuff = zeros(4,8);
    LQE_Z_spuff = satInfo;
    
%     for ii = 1:corruptSatCount
    psdRange_spuff(1:corruptSatCount) = psdRange_spuff(corruptSatCount)   + errVal;
    LQE_Z_spuff(2,1:corruptSatCount)  = LQE_Z_spuff(2,corruptSatCount)    + errVal;
%     end
    
%     if errVal ~= 0 
%             qqq = 1;
%     end
%     
    if ctrlSatCoefs == 1
        for ii = 1:3
            jj = find(satInctrl(ii) == satID);
            psdRange_spuff(jj) = psdRange_spuff(jj) - satCoefs(1,ii) - satCoefs(2,ii) * satCoefs(4,ii) - satCoefs(3,ii) * satCoefs(4,ii).^2;
            LQE_Z_spuff(2,jj)  = LQE_Z_spuff(2,jj)  - satCoefs(1,ii) - satCoefs(2,ii) * satCoefs(4,ii) - satCoefs(3,ii) * satCoefs(4,ii).^2;
        end
    end
%     jj = satPunishableID;%find(satPunishableID == satID);
%     
%     psdRange_spuff(1:3) = psdRange_spuff(1:3)   + errVal;
%     LQE_Z_spuff(2,1:3)  = LQE_Z_spuff(2,1:3)    + errVal;
%     
%     psdRange_spuff(jj) = psdRange_spuff(jj)   + errVal;
%     LQE_Z_spuff(2,jj)  = LQE_Z_spuff(2,jj)    + errVal;
    
%     for ii = 1:3
%         jj = find(satInctrl(ii) == satID);
%         psdRange_spuff(jj) = psdRange_spuff(jj) - satCoefs(1,ii) - satCoefs(2,ii) * satCoefs(4,ii) - satCoefs(3,ii) * satCoefs(4,ii).^2;
%         LQE_Z_spuff(2,jj)  = LQE_Z_spuff(2,jj)  - satCoefs(1,ii) - satCoefs(2,ii) * satCoefs(4,ii) - satCoefs(3,ii) * satCoefs(4,ii).^2;
%     end
    
end

function result = find_(data, array)

    for ii = 1:length(array)
        if array(ii) == data
            result = ii;
        end
    end

end

function [result, count] = findAll_(data, array) 
    result = zeros(size(array));
    count  = 0;
    
    for ii = 1:length(array)
        if array(ii) == data
            count         = count + 1;
            result(count) = count;
        end
    end
end

== matlab function base_model_lqeH/seter3 ==
  data: signal output size=1; time_shift input
function signal  = slowData(time_shift)
  
    persistent time_mem

    if isempty(time_mem)
        time_mem = 0;
    end
    
    signal = 0;
    time_mem = time_mem + time_shift;
    
    if time_mem >= 1
        signal = 1;
        time_mem = 0;
    end
    
end

== matlab function base_model_lqeH/seter4 ==
  data: signal output size=1; time_shift input
function signal  = slowData(time_shift)
  
    persistent time_mem

    if isempty(time_mem)
        time_mem = 0;
    end
    
    signal = 0;
    time_mem = time_mem + time_shift;
    
    if time_mem >= 1
        signal = 1;
        time_mem = 0;
    end
    
end

== matlab function base_model_lqeH/seter5 ==
  data: signal output size=1; time_shift input
function signal  = slowData(time_shift)
  
    persistent time_mem

    if isempty(time_mem)
        time_mem = 0;
    end
    
    signal = 0;
    time_mem = time_mem + time_shift;
    
    if time_mem >= 1
        signal = 1;
        time_mem = 0;
    end
    
end

== matlab function base_model_lqeH/seter10 ==
  data: signal output size=1; time_shift input
function signal  = slowData(time_shift)
  
    persistent time_mem

    if isempty(time_mem)
        time_mem = 0;
    end
    
    signal = 0;
    time_mem = time_mem + time_shift;
    
    if time_mem >= 1
        signal = 1;
        time_mem = 0;
    end
    
end

== matlab function base_model_lqeH/Fuck matlab2 ==
  data: data_fix output size=8; data input; criteria input; satCountPreset input
function data_fix =  forCtrl(data, criteria, satCountPreset)
    
    data_fix = zeros(8,1);
    for ii = 1:8
        if data(ii) > criteria
            data(ii) = nan;
        end
    end
    data_fix = data;    
end

== matlab function base_model_lqeH/seter6 ==
  data: signal output size=1; time_shift input
function signal  = slowData(time_shift)
  
    persistent time_mem

    if isempty(time_mem)
        time_mem = 0;
    end
    
    signal = 0;
    time_mem = time_mem + time_shift;
    
    if time_mem >= 1
        signal = 1;
        time_mem = 0;
    end
    
end

== matlab function base_model_lqeH/seter7 ==
  data: signal output size=1; time_shift input
function signal  = slowData(time_shift)
  
    persistent time_mem

    if isempty(time_mem)
        time_mem = 0;
    end
    
    signal = 0;
    time_mem = time_mem + time_shift;
    
    if time_mem >= 1
        signal = 1;
        time_mem = 0;
    end
    
end

== matlab function base_model_lqeH/seter8 ==
  data: signal output size=1; time_shift input
function signal  = slowData(time_shift)
  
    persistent time_mem

    if isempty(time_mem)
        time_mem = 0;
    end
    
    signal = 0;
    time_mem = time_mem + time_shift;
    
    if time_mem >= 1
        signal = 1;
        time_mem = 0;
    end
    
end

== matlab function base_model_lqeH/seter9 ==
  data: signal output size=1; time_shift input
function signal  = slowData(time_shift)
  
    persistent time_mem

    if isempty(time_mem)
        time_mem = 0;
    end
    
    signal = 0;
    time_mem = time_mem + time_shift;
    
    if time_mem >= 1
        signal = 1;
        time_mem = 0;
    end
    
end
